simulink model "clothoidSimulation1"  (R2013a)
settings: Solver=ode45  StartTime=0.0  StopTime=S  MaxStep=.1  RelTol=1e-3
undefined symbols (not defined in the file or in its folder): kA, kB, PS, S, thetaS
settings Model: Creator=klaus  LastModifiedBy=KWS

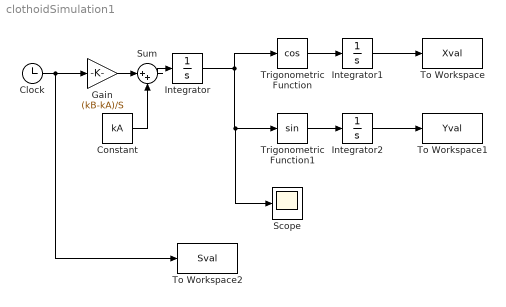
== system clothoidSimulation1 ==
  Clock : Clock
  Constant : Constant  Value=kA
  Gain : Gain  Gain=(kB-kA)/S
  Integrator : Integrator  InitialCondition=thetaS
  Integrator1 : Integrator  InitialCondition=PS(1)
  Integrator2 : Integrator  InitialCondition=PS(2)
  Scope : Scope
  Sum : Sum  Inputs=|++
  To Workspace : ToWorkspace  VariableName=Xval  SampleTime=-1
  To Workspace1 : ToWorkspace  VariableName=Yval  SampleTime=-1
  To Workspace2 : ToWorkspace  VariableName=Sval  SampleTime=-1
  Trigonometric Function : Trigonometry  Operator=cos
  Trigonometric Function1 : Trigonometry
  wires:
  Clock/1 -> To Workspace2/1, Gain/1
  Integrator/1 -> Scope/1, Trigonometric Function1/1, Trigonometric Function/1
  Trigonometric Function/1 -> Integrator1/1
  Trigonometric Function1/1 -> Integrator2/1
  Integrator1/1 -> To Workspace/1
  Integrator2/1 -> To Workspace1/1
  Sum/1 -> Integrator/1
  Gain/1 -> Sum/1
  Constant/1 -> Sum/2
